simulink model "schema_slaba"  (R2024b)
settings: Solver=VariableStepAuto  StartTime=0.0  StopTime=0.2  MaxStep=1e-3  RelTol=1e-3
values from neighbouring files (symbols this model uses):
  CA0 = CA02    [Slaba_verzia.m]
  CAf = input('Zadaj CAf [mol/l]:')    [Slaba_verzia.m]
  CB0 = k1*CA0/(k2+F0/V)    [Slaba_verzia.m]
  F0 = input('Zadaj F0 [l/h]:')    [Slaba_verzia.m]
  P_z = conv([1 -1], [p0_0_value p0_1_value] )    [Slaba_verzia.m]
  Q_z = (q0_0_value) * A_plus    [Slaba_verzia.m]
  T = ((1/10) * t_ust)    [Slaba_verzia.m]
settings Model: Creator=gchuc  LastModifiedBy=glebe

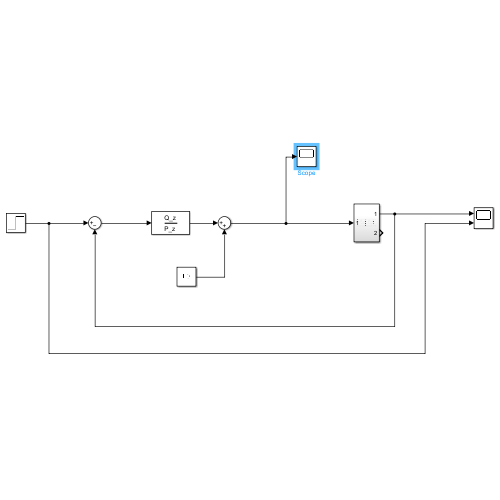
[thumbnail: Simulink's stored preview of the top-level diagram]
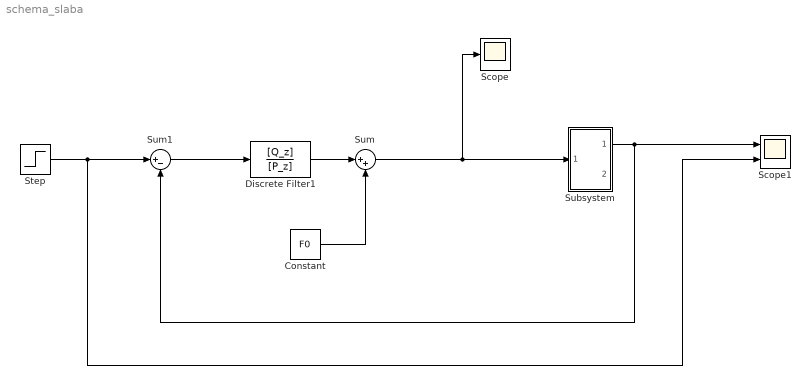
== system schema_slaba ==
  Constant : Constant  Value=F0
  Discrete Filter1 : DiscreteFilter  Numerator=[Q_z]  Denominator=[P_z]  SampleTime=T
  Scope : Scope
  Scope1 : Scope  NumInputPorts=2
  Step : Step  Time=0.1  Before=CB0  After=CB0+0.0016  SampleTime=0
  Subsystem : Subsystem
  Sum : Sum  Inputs=|++
  Sum1 : Sum  Inputs=|+-
  wires:
  Step/1 -> Scope1/2, Sum1/1
  Constant/1 -> Sum/2
  Sum/1 -> Scope/1, Subsystem/1(In1)
  Sum1/1 -> Discrete Filter1/1
  Discrete Filter1/1 -> Sum/1
  Subsystem/1(Out2) -> Scope1/1, Sum1/2

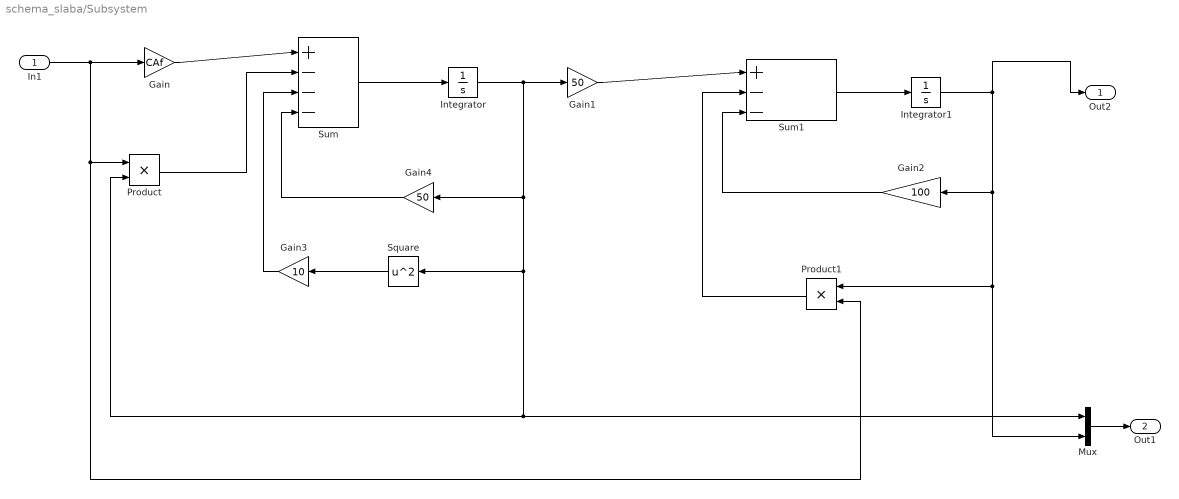
== system schema_slaba/Subsystem ==
  In1 : Inport
  Gain : Gain  Gain=CAf
  Gain1 : Gain  Gain=50
  Gain2 : Gain  Gain=100
  Gain3 : Gain  Gain=10
  Gain4 : Gain  Gain=50
  Integrator : Integrator  InitialCondition=CA0
  Integrator1 : Integrator  InitialCondition=CB0
  Mux : Mux  Inputs=2
  Product : Product
  Product1 : Product
  Square : Math  Operator=square
  Sum : Sum  Inputs=|+---
  Sum1 : Sum  Inputs=|+--
  Out2 : Outport
  Out1 : Outport  Port=2
  wires:
  Integrator/1 -> Gain4/1, Square/1, Mux/1, Product/2, Gain1/1
  Gain1/1 -> Sum1/1
  In1/1 -> Product1/2, Product/1, Gain/1
  Integrator1/1 -> Out2/1, Mux/2, Product1/1, Gain2/1
  Gain3/1 -> Sum/3
  Gain/1 -> Sum/1
  Sum/1 -> Integrator/1
  Product/1 -> Sum/2
  Gain2/1 -> Sum1/3
  Product1/1 -> Sum1/2
  Sum1/1 -> Integrator1/1
  Mux/1 -> Out1/1
  Square/1 -> Gain3/1
  Gain4/1 -> Sum/4
